simulink model "Bernoullis_Eq_Sim"  (R2024b)
settings: Solver=VariableStepAuto  StartTime=0.0  StopTime=10.0  RelTol=1e-3
undefined symbols (not defined in the file or in its folder): P1_Pa, p_kgpm3, V1_mps, V2_mps
settings Model: Creator=Stephon Woodson  LastModifiedBy=Stephon Woodson

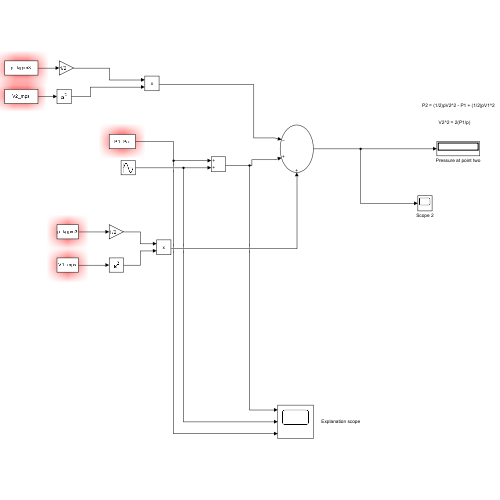
[thumbnail: Simulink's stored preview of the top-level diagram]
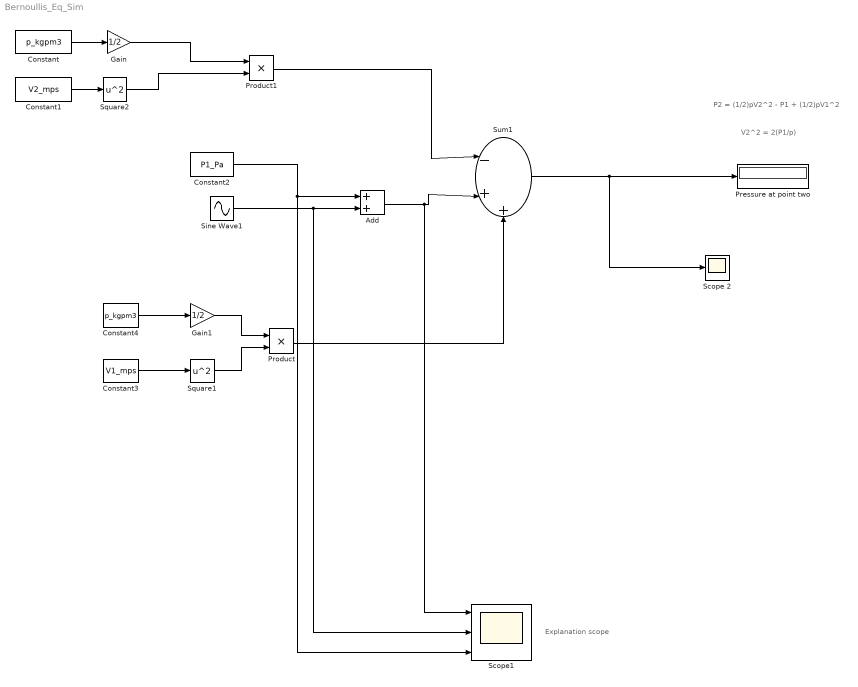
== system Bernoullis_Eq_Sim ==
  note: P2 = (1/2)pV2^2 - P1 + (1/2)pV1^2
  note: V2^2 = 2(P1/p)
  note: Explanation scope
  Add : Sum
  Constant : Constant  Value=p_kgpm3
  Constant1 : Constant  Value=V2_mps
  Constant2 : Constant  Value=P1_Pa
  Constant3 : Constant  Value=V1_mps
  Constant4 : Constant  Value=p_kgpm3
  Gain : Gain  Gain=1/2
  Gain1 : Gain  Gain=1/2
  Pressure at point two : Display
  Product : Product
  Product1 : Product
  Scope 2 : Scope
  Scope1 : Scope  NumInputPorts=3
  Sine Wave1 : Sin  SampleTime=0
  Square1 : Math  Operator=square
  Square2 : Math  Operator=square
  Sum1 : Sum  Inputs=|-++
  wires:
  Gain1/1 -> Product/1
  Square2/1 -> Product1/2
  Sum1/1 -> Scope 2/1, Pressure at point two/1
  Sine Wave1/1 -> Scope1/2, Add/2
  Product1/1 -> Sum1/1
  Constant4/1 -> Gain1/1
  Constant1/1 -> Square2/1
  Add/1 -> Scope1/1, Sum1/2
  Constant2/1 -> Scope1/3, Add/1
  Constant/1 -> Gain/1
  Product/1 -> Sum1/3
  Gain/1 -> Product1/1
  Square1/1 -> Product/2
  Constant3/1 -> Square1/1
